simulink library "SUB_ECU_L4_MABX"  (R2018a)
settings: Solver=VariableStepAuto  StartTime=0.0  StopTime=10.0  RelTol=1e-3
libraries: EmE_MBD_Blockset x76, simulink x14, SUB_L4_Task_10000ms x1, SUB_L4_Task_1000ms x1, SUB_L4_Task_100ms x1, SUB_L4_Task_10ms_SUB_APTC x1, PTC_MBDS_LIB x1, SUB_L4_Task_10ms_SUB_BRKPEDARB x1, SUB_L4_Task_10ms_SUB_FAULT_MANAGER x1, SUB_L4_Task_10ms_SUB_STATE_CONTROL x1, SUB_L4_Task_10ms_SUB_STEERCTRL x1, simulink_need_slupdate x1
(part 1 of 2)
settings Model: Creator=Chris.Balton  LastModifiedBy=Gavin.Coelho

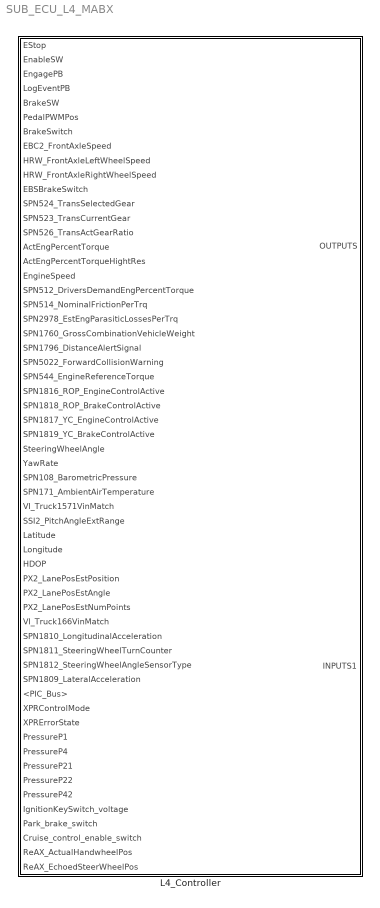
== system SUB_ECU_L4_MABX ==
  L4_Controller : Subsystem

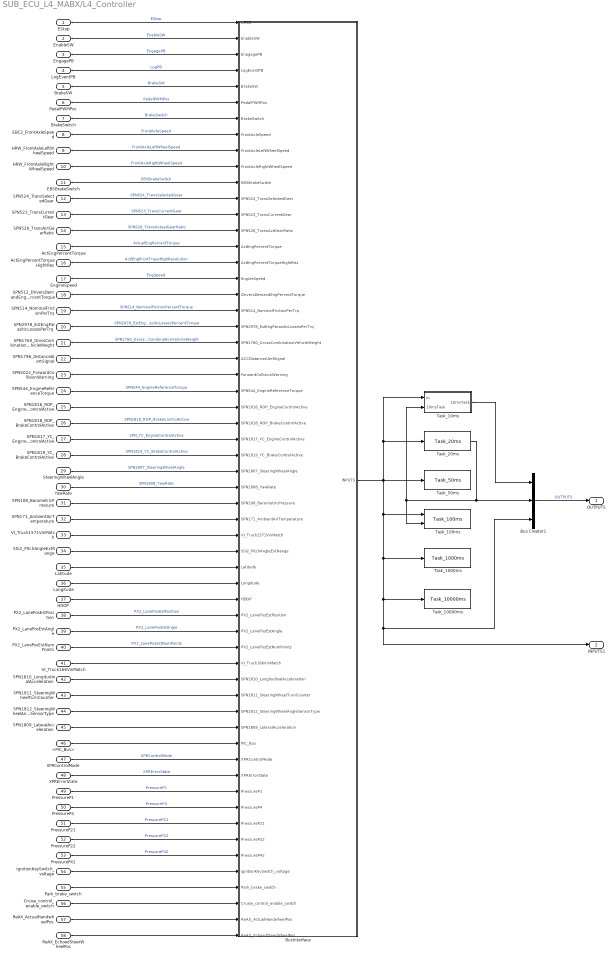
== system SUB_ECU_L4_MABX/L4_Controller ==
  EStop : Inport
  EnableSW : Inport  Port=2
  EngagePB : Inport  Port=3
  LogEventPB : Inport  Port=4
  BrakeSW : Inport  Port=5
  PedalPWMPos : Inport  Port=6
  BrakeSwitch : Inport  Port=7
  EBC2_FrontAxleSpeed : Inport  Port=8
  HRW_FrontAxleLeftWheelSpeed : Inport  Port=9
  HRW_FrontAxleRightWheelSpeed : Inport  Port=10
  EBSBrakeSwitch : Inport  Port=11
  SPN524_TransSelectedGear : Inport  Port=12
  SPN523_TransCurrentGear : Inport  Port=13
  SPN526_TransActGearRatio : Inport  Port=14
  ActEngPercentTorque : Inport  Port=15
  ActEngPercentTorqueHightRes : Inport  Port=16
  EngineSpeed : Inport  Port=17
  SPN512_DriversDemandEngPercentTorque : Inport  Port=18
  SPN514_NominalFrictionPerTrq : Inport  Port=19
  SPN2978_EstEngParasiticLossesPerTrq : Inport  Port=20
  SPN1760_GrossCombinationVehicleWeight : Inport  Port=21
  SPN1796_DistanceAlertSignal : Inport  Port=22
  SPN5022_ForwardCollisionWarning : Inport  Port=23
  SPN544_EngineReferenceTorque : Inport  Port=24
  SPN1816_ROP_EngineControlActive : Inport  Port=25
  SPN1818_ROP_BrakeControlActive : Inport  Port=26
  SPN1817_YC_EngineControlActive : Inport  Port=27
  SPN1819_YC_BrakeControlActive : Inport  Port=28
  SteeringWheelAngle : Inport  Port=29
  YawRate : Inport  Port=30
  SPN108_BarometricPressure : Inport  Port=31
  SPN171_AmbientAirTemperature : Inport  Port=32
  VI_Truck1571VinMatch : Inport  Port=33
  SSI2_PitchAngleExtRange : Inport  Port=34
  Latitude : Inport  Port=35
  Longitude : Inport  Port=36
  HDOP : Inport  Port=37
  PX2_LanePosEstPosition : Inport  Port=38
  PX2_LanePosEstAngle : Inport  Port=39
  PX2_LanePosEstNumPoints : Inport  Port=40
  VI_Truck166VinMatch : Inport  Port=41
  SPN1810_LongitudinalAcceleration : Inport  Port=42
  SPN1811_SteeringWheelTurnCounter : Inport  Port=43
  SPN1812_SteeringWheelAngleSensorType : Inport  Port=44
  SPN1809_LateralAcceleration : Inport  Port=45
  <PIC_Bus> : Inport  Port=46
  XPRControlMode : Inport  Port=47
  XPRErrorState : Inport  Port=48
  PressureP1 : Inport  Port=49
  PressureP4 : Inport  Port=50
  PressureP21 : Inport  Port=51
  PressureP22 : Inport  Port=52
  PressureP42 : Inport  Port=53
  IgnitionKeySwitch_voltage : Inport  Port=54
  Park_brake_switch : Inport  Port=55
  Cruise_control_enable_switch : Inport  Port=56
  ReAX_ActualHandwheelPos : Inport  Port=57
  ReAX_EchoedSteerWheelPos : Inport  Port=58
  Bus Creator1 : BusCreator  Inputs=3
  BusInterface : Subsystem
  Task_10000ms : SUB_L4_Task_10000ms/Task_10000ms
  Task_1000ms : SUB_L4_Task_1000ms/Task_1000ms
  Task_100ms : SUB_L4_Task_100ms/Task_100ms
  Task_10ms : Subsystem  TreatAsAtomicUnit=on  SystemSampleTime=0.01
  Task_20ms : SUB_L4_Task_20ms/Task_20ms
  Task_50ms : SUB_L4_Task_50ms/Task_50ms
  OUTPUTS : Outport
  INPUTS1 : Outport  Port=2
  wires:
  BrakeSW/1 -> BusInterface/5(BrakeSW)  "BrakeSW"
  ReAX_EchoedSteerWheelPos/1 -> BusInterface/58(ReAX_EchoedSteerWheelPos)
  ReAX_ActualHandwheelPos/1 -> BusInterface/57(ReAX_ActualHandwheelPos)
  EngagePB/1 -> BusInterface/3(EnagagePB)  "EngagePB"
  SPN1809_LateralAcceleration/1 -> BusInterface/45(SPN1809_LateralAcceleration)
  XPRErrorState/1 -> BusInterface/48(XPRErrorState)  "XPRErrorState"
  PressureP1/1 -> BusInterface/49(PressureP1)  "PressureP1"
  PressureP4/1 -> BusInterface/50(PressureP4)  "PressureP4"
  PressureP21/1 -> BusInterface/51(PressureP21)  "PressureP21"
  EBC2_FrontAxleSpeed/1 -> BusInterface/8(FrontAxleSpeed)  "FrontAxleSpeed"
  Task_10ms/1(10msTask) -> Bus Creator1/1
  EngineSpeed/1 -> BusInterface/17(EngineSpeed)  "EngSpeed"
  Cruise_control_enable_switch/1 -> BusInterface/56(Cruise_control_enable_switch)
  Longitude/1 -> BusInterface/36(Longitude)
  SPN5022_ForwardCollisionWarning/1 -> BusInterface/23(ForwardCollisionWarning)
  VI_Truck1571VinMatch/1 -> BusInterface/33(VI_Truck1571VinMatch)
  SPN512_DriversDemandEngPercentTorque/1 -> BusInterface/18(DriversDemandEngPercentTorque)
  Task_20ms/1 -> Bus Creator1/2, Task_100ms/2, Task_10ms/2(20msTask)
  SPN171_AmbientAirTemperature/1 -> BusInterface/32(SPN171_AmbientAirTemperature)
  SPN544_EngineReferenceTorque/1 -> BusInterface/24(SPN544_EngineReferenceTorque)  "SPN544_EngineReferenceTorque"
  HRW_FrontAxleRightWheelSpeed/1 -> BusInterface/10(FrontAxleRightWheelSpeed)  "FrontAxleRightWheelSpeed"
  SPN108_BarometricPressure/1 -> BusInterface/31(SPN108_BarometricPressure)
  PedalPWMPos/1 -> BusInterface/6(PedalPWMPos)  "PedalPWMPos"
  SPN524_TransSelectedGear/1 -> BusInterface/12(SPN524_TransSelectedGear)  "SPN524_TransSelectedGear"
  SPN1796_DistanceAlertSignal/1 -> BusInterface/22(ACCDistanceAlertSignal)
  Bus Creator1/1 -> OUTPUTS/1  "OUTPUTS"
  SPN1819_YC_BrakeControlActive/1 -> BusInterface/28(SPN1819_YC_BrakeControlActive)  "SPN1819_YC_BrakeControlActive"
  ActEngPercentTorque/1 -> BusInterface/15(ActEngPercentTorque)  "ActualEngPercentTorque"
  XPRControlMode/1 -> BusInterface/47(XPRControlMode)  "XPRControlMode"
  SSI2_PitchAngleExtRange/1 -> BusInterface/34(SSI2_PitchAngleExtRange)
  IgnitionKeySwitch_voltage/1 -> BusInterface/54(IgnitionKeySwitch_voltage)
  BrakeSwitch/1 -> BusInterface/7(BrakeSwitch)  "BrakeSwitch"
  HRW_FrontAxleLeftWheelSpeed/1 -> BusInterface/9(FrontAxleLeftWheelSpeed)  "FrontAxleLeftWheelSpeed"
  BusInterface/1(INPUTS) -> Task_50ms/1, Task_20ms/1, Task_10ms/1(In), Task_100ms/1, Task_1000ms/1, Task_10000ms/1, Bus Creator1/3, INPUTS1/1
  Park_brake_switch/1 -> BusInterface/55(Park_brake_switch)
  <PIC_Bus>/1 -> BusInterface/46(PIC_Bus)
  Latitude/1 -> BusInterface/35(Latitude)
  PressureP22/1 -> BusInterface/52(PressureP22)  "PressureP22"
  PressureP42/1 -> BusInterface/53(PressureP42)  "PressureP42"
  PX2_LanePosEstPosition/1 -> BusInterface/38(PX2_LanePosEstPosition)  "PX2_LanePosEstPosition"
  SPN514_NominalFrictionPerTrq/1 -> BusInterface/19(SPN514_NominalFrictionPerTrq)  "SPN514_NominalFrictionPercentTorque"
  SteeringWheelAngle/1 -> BusInterface/29(SPN1807_SteeringWheelAngle)  "SPN1807_SteeringWheelAngle"
  HDOP/1 -> BusInterface/37(HDOP)
  YawRate/1 -> BusInterface/30(SPN1808_YawRate)  "SPN1808_YawRate"
  EBSBrakeSwitch/1 -> BusInterface/11(EBSBrakeSwitch)  "EBSBrakeSwitch"
  SPN1811_SteeringWheelTurnCounter/1 -> BusInterface/43(SPN1811_SteeringWheelTurnCounter)
  SPN1760_GrossCombinationVehicleWeight/1 -> BusInterface/21(SPN1760_GrossCombinationVehicleWeight)  "SPN1760_GrossCombinationVehicleWeight"
  SPN2978_EstEngParasiticLossesPerTrq/1 -> BusInterface/20(SPN2978_EstEngParasiticLossesPerTrq)  "SPN2978_EstEngParasiticLossesPercentTorque"
  SPN1812_SteeringWheelAngleSensorType/1 -> BusInterface/44(SPN1812_SteeringWheelAngleSensorType)
  SPN526_TransActGearRatio/1 -> BusInterface/14(SPN526_TransActGearRatio)  "SPN526_TransActualGearRatio"
  SPN1818_ROP_BrakeControlActive/1 -> BusInterface/26(SPN1818_ROP_BrakeControlActive)  "SPN1818_ROP_BrakeControlActive"
  PX2_LanePosEstAngle/1 -> BusInterface/39(PX2_LanePosEstAngle)  "PX2_LanePosEstAngle"
  ActEngPercentTorqueHightRes/1 -> BusInterface/16(ActEngPercentTorqueHightRes)  "ActlEngPrcntTrqueHighResolution"
  SPN1810_LongitudinalAcceleration/1 -> BusInterface/42(SPN1810_LongitudinalAcceleration)
  PX2_LanePosEstNumPoints/1 -> BusInterface/40(PX2_LanePosEstNumPoints)  "PX2_LanePosEstNumPoints"
  EStop/1 -> BusInterface/1(Estop)  "EStop"
  VI_Truck166VinMatch/1 -> BusInterface/41(VI_Truck166VinMatch)
  SPN523_TransCurrentGear/1 -> BusInterface/13(SPN523_TransCurrentGear)  "SPN523_TransCurrentGear"
  SPN1817_YC_EngineControlActive/1 -> BusInterface/27(SPN1817_YC_EngineControlActive)  "SPN_YC_EngineControlActive"
  EnableSW/1 -> BusInterface/2(EnableSW)  "EnableSW"
  SPN1816_ROP_EngineControlActive/1 -> BusInterface/25(SPN1816_ROP_EngineControlActive)
  LogEventPB/1 -> BusInterface/4(LogEventPB)  "LogPB"

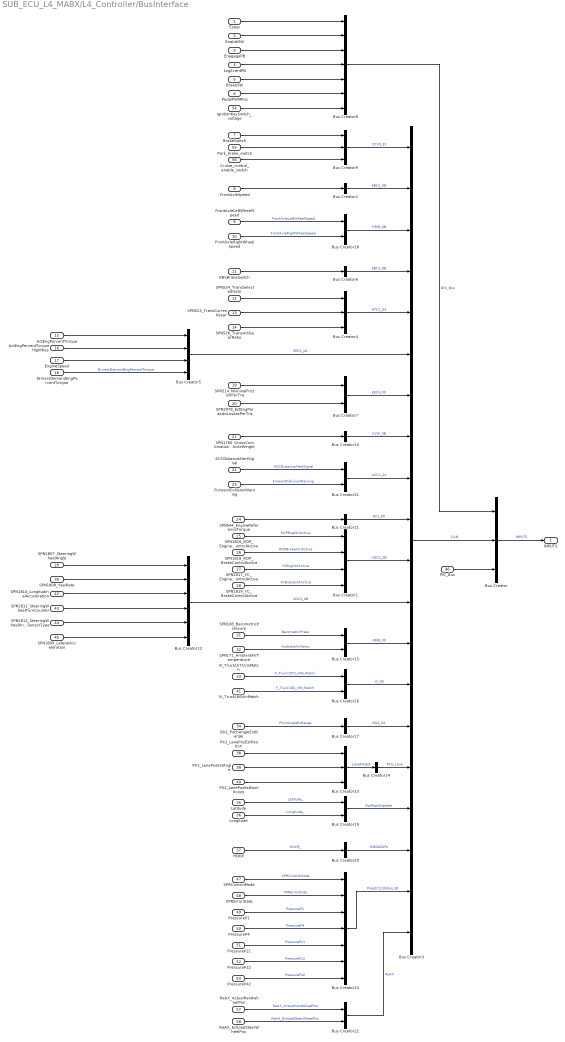
== system SUB_ECU_L4_MABX/L4_Controller/BusInterface ==
  Estop : Inport
  EnableSW : Inport  Port=2
  EnagagePB : Inport  Port=3
  LogEventPB : Inport  Port=4
  BrakeSW : Inport  Port=5
  PedalPWMPos : Inport  Port=6
  BrakeSwitch : Inport  Port=7
  FrontAxleSpeed : Inport  Port=8
  FrontAxleLeftWheelSpeed : Inport  Port=9
  FrontAxleRightWheelSpeed : Inport  Port=10
  EBSBrakeSwitch : Inport  Port=11
  SPN524_TransSelectedGear : Inport  Port=12
  SPN523_TransCurrentGear : Inport  Port=13
  SPN526_TransActGearRatio : Inport  Port=14
  ActEngPercentTorque : Inport  Port=15
  ActEngPercentTorqueHightRes : Inport  Port=16
  EngineSpeed : Inport  Port=17
  DriversDemandEngPercentTorque : Inport  Port=18
  SPN514_NominalFrictionPerTrq : Inport  Port=19
  SPN2978_EstEngParasiticLossesPerTrq : Inport  Port=20
  SPN1760_GrossCombinationVehicleWeight : Inport  Port=21
  ACCDistanceAlertSignal : Inport  Port=22
  ForwardCollisionWarning : Inport  Port=23
  SPN544_EngineReferenceTorque : Inport  Port=24
  SPN1816_ROP_EngineControlActive : Inport  Port=25
  SPN1818_ROP_BrakeControlActive : Inport  Port=26
  SPN1817_YC_EngineControlActive : Inport  Port=27
  SPN1819_YC_BrakeControlActive : Inport  Port=28
  SPN1807_SteeringWheelAngle : Inport  Port=29
  SPN1808_YawRate : Inport  Port=30
  SPN108_BarometricPressure : Inport  Port=31
  SPN171_AmbientAirTemperature : Inport  Port=32
  VI_Truck1571VinMatch : Inport  Port=33
  SSI2_PitchAngleExtRange : Inport  Port=34
  Latitude : Inport  Port=35
  Longitude : Inport  Port=36
  HDOP : Inport  Port=37
  PX2_LanePosEstPosition : Inport  Port=38
  PX2_LanePosEstAngle : Inport  Port=39
  PX2_LanePosEstNumPoints : Inport  Port=40
  VI_Truck166VinMatch : Inport  Port=41
  SPN1810_LongitudinalAcceleration : Inport  Port=42
  SPN1811_SteeringWheelTurnCounter : Inport  Port=43
  SPN1812_SteeringWheelAngleSensorType : Inport  Port=44
  SPN1809_LateralAcceleration : Inport  Port=45
  PIC_Bus : Inport  Port=46
  XPRControlMode : Inport  Port=47
  XPRErrorState : Inport  Port=48
  PressureP1 : Inport  Port=49
  PressureP4 : Inport  Port=50
  PressureP21 : Inport  Port=51
  PressureP22 : Inport  Port=52
  PressureP42 : Inport  Port=53
  IgnitionKeySwitch_voltage : Inport  Port=54
  Park_brake_switch : Inport  Port=55
  Cruise_control_enable_switch : Inport  Port=56
  ReAX_ActualHandwheelPos : Inport  Port=57
  ReAX_EchoedSteerWheelPos : Inport  Port=58
  Bus Creator{,4,9,13} (4 alike) : BusCreator  Inputs=3
  Bus Creator1 : BusCreator  Inputs=4
  Bus Creator{2,6,10..11,14,17,20} (7 alike) : BusCreator  Inputs=1
  Bus Creator12 : BusCreator  Inputs=6
  Bus Creator{7,15..16,18..19,21..22} (7 alike) : BusCreator  Inputs=2
  Bus Creator23 : BusCreator  Inputs=7
  Bus Creator3 : BusCreator  Inputs=20
  Bus Creator5 : BusCreator  Inputs=4
  Bus Creator8 : BusCreator  Inputs=7
  INPUTS : Outport
  wires:
  BrakeSW/1 -> Bus Creator8/5
  Bus Creator22/1 -> Bus Creator3/20  "ReAX"
  ReAX_ActualHandwheelPos/1 -> Bus Creator22/1  "ReAX_ActualHandwheelPos"
  ReAX_EchoedSteerWheelPos/1 -> Bus Creator22/2  "ReAX_EchoedSteerWheelPos"
  Bus Creator23/1 -> Bus Creator3/19  "Prop2C2_Status_30"
  XPRControlMode/1 -> Bus Creator23/1  "XPRControlMode"
  PressureP21/1 -> Bus Creator23/5  "PressureP21"
  XPRErrorState/1 -> Bus Creator23/2  "XPRErrorState"
  PressureP42/1 -> Bus Creator23/7  "PressureP42"
  PressureP1/1 -> Bus Creator23/3  "PressureP1"
  PressureP22/1 -> Bus Creator23/6  "PressureP22"
  PressureP4/1 -> Bus Creator23/4  "PressureP4"
  SPN1809_LateralAcceleration/1 -> Bus Creator12/6
  SPN1812_SteeringWheelAngleSensorType/1 -> Bus Creator12/5
  SPN1811_SteeringWheelTurnCounter/1 -> Bus Creator12/4
  SPN1810_LongitudinalAcceleration/1 -> Bus Creator12/3
  VI_Truck166VinMatch/1 -> Bus Creator16/2  "F_Truck166_VIN_Match"
  Bus Creator1/1 -> Bus Creator3/11  "VDC1_0B"
  SPN1819_YC_BrakeControlActive/1 -> Bus Creator1/4  "YCBrakeCtrlActive"
  SPN1817_YC_EngineControlActive/1 -> Bus Creator1/3  "YCEngCtrlActive"
  SPN1818_ROP_BrakeControlActive/1 -> Bus Creator1/2  "ROPBrakeCtrlActive"
  SPN1816_ROP_EngineControlActive/1 -> Bus Creator1/1  "ROPEngCtrlActive"
  SPN1808_YawRate/1 -> Bus Creator12/2
  Bus Creator/1 -> INPUTS/1  "INPUTS"
  EngineSpeed/1 -> Bus Creator5/3
  PX2_LanePosEstPosition/1 -> Bus Creator13/1
  FrontAxleSpeed/1 -> Bus Creator2/1
  SPN1807_SteeringWheelAngle/1 -> Bus Creator12/1
  Bus Creator14/1 -> Bus Creator3/16  "PX2_Lane"
  SPN526_TransActGearRatio/1 -> Bus Creator4/3
  SPN544_EngineReferenceTorque/1 -> Bus Creator11/1
  Bus Creator12/1 -> Bus Creator3/12  "VDC2_0B"
  Bus Creator6/1 -> Bus Creator3/4  "EBC1_0B"
  Bus Creator4/1 -> Bus Creator3/5  "ETC2_03"
  SPN2978_EstEngParasiticLossesPerTrq/1 -> Bus Creator7/2
  SPN514_NominalFrictionPerTrq/1 -> Bus Creator7/1
  SPN524_TransSelectedGear/1 -> Bus Creator4/1
  Bus Creator2/1 -> Bus Creator3/2  "EBC2_0B"
  SPN523_TransCurrentGear/1 -> Bus Creator4/2
  Bus Creator9/1 -> Bus Creator3/1  "CCVS_31"
  Bus Creator10/1 -> Bus Creator3/8  "CVW_0B"
  PX2_LanePosEstAngle/1 -> Bus Creator13/2
  SPN1760_GrossCombinationVehicleWeight/1 -> Bus Creator10/1
  Bus Creator7/1 -> Bus Creator3/7  "EEC3_00"
  ActEngPercentTorqueHightRes/1 -> Bus Creator5/2
  Bus Creator11/1 -> Bus Creator3/10  "EC1_00"
  EBSBrakeSwitch/1 -> Bus Creator6/1
  BrakeSwitch/1 -> Bus Creator9/1
  Bus Creator3/1 -> Bus Creator/2  "CAN"
  ActEngPercentTorque/1 -> Bus Creator5/1
  EnagagePB/1 -> Bus Creator8/3
  Bus Creator5/1 -> Bus Creator3/6  "EEC1_00"
  PX2_LanePosEstNumPoints/1 -> Bus Creator13/3
  Bus Creator8/1 -> Bus Creator/1  "DIO_Bus"
  Bus Creator13/1 -> Bus Creator14/1  "LanePosEst"
  SPN108_BarometricPressure/1 -> Bus Creator15/1  "BarometricPress"
  SPN171_AmbientAirTemperature/1 -> Bus Creator15/2  "AmbientAirTemp"
  VI_Truck1571VinMatch/1 -> Bus Creator16/1  "F_Truck1571_VIN_Match"
  SSI2_PitchAngleExtRange/1 -> Bus Creator17/1  "PitchAngleExRange"
  Bus Creator15/1 -> Bus Creator3/13  "AMB_00"
  Bus Creator16/1 -> Bus Creator3/14  "VI_00"
  Bus Creator17/1 -> Bus Creator3/15  "SSI2_03"
  PedalPWMPos/1 -> Bus Creator8/6
  FrontAxleLeftWheelSpeed/1 -> Bus Creator18/1  "FrontAxleLeftWheelSpeed"
  FrontAxleRightWheelSpeed/1 -> Bus Creator18/2  "FrontAxleRightWheelSpeed"
  Bus Creator18/1 -> Bus Creator3/3  "HRW_0B"
  Latitude/1 -> Bus Creator19/1  "Latitude_"
  Longitude/1 -> Bus Creator19/2  "Longitude_"
  Bus Creator19/1 -> Bus Creator3/17  "PosRapidUpdate"
  HDOP/1 -> Bus Creator20/1  "HDOP_"
  Bus Creator20/1 -> Bus Creator3/18  "GNSSDOPs"
  ACCDistanceAlertSignal/1 -> Bus Creator21/1  "ACCDistanceAlertSignal"
  ForwardCollisionWarning/1 -> Bus Creator21/2  "ForwardCollisionWarning"
  Bus Creator21/1 -> Bus Creator3/9  "ACC1_2A"
  DriversDemandEngPercentTorque/1 -> Bus Creator5/4  "DriversDemandEngPercentTorque"
  PIC_Bus/1 -> Bus Creator/3
  IgnitionKeySwitch_voltage/1 -> Bus Creator8/7
  Park_brake_switch/1 -> Bus Creator9/2
  Cruise_control_enable_switch/1 -> Bus Creator9/3
  EnableSW/1 -> Bus Creator8/2
  Estop/1 -> Bus Creator8/1
  LogEventPB/1 -> Bus Creator8/4

== system SUB_ECU_L4_MABX/L4_Controller/Task_10ms ==
  In : Inport
  20msTask : Inport  Port=2
  APTC_10ms : SUB_L4_Task_10ms_SUB_APTC/APTC_10ms
  AutonomousEnable : Subsystem
  BRKPEDARB_10ms : SUB_L4_Task_10ms_SUB_BRKPEDARB/BRKPEDARB_10ms
  Bus Creator : BusCreator  Inputs=6
  FAULT_MANAGER_10ms : SUB_L4_Task_10ms_SUB_FAULT_MANAGER/FAULT_MANAGER_10ms
  STATE_CONTROL_10ms : SUB_L4_Task_10ms_SUB_STATE_CONTROL/STATE_CONTROL_10ms
  STEERCTRL_10ms : SUB_L4_Task_10ms_SUB_STEERCTRL/STEERCTRL_10ms
  Vehicle_speed_target : Subsystem
  10msTask : Outport
  wires:
  In/1 -> AutonomousEnable/1(In)
  APTC_10ms/1 -> Bus Creator/2  "APTC"
  Bus Creator/1 -> 10msTask/1  "10msTask"
  STEERCTRL_10ms/1 -> STATE_CONTROL_10ms/3, BRKPEDARB_10ms/2, Bus Creator/1  "SteeringControl"
  STATE_CONTROL_10ms/1 -> Bus Creator/3, APTC_10ms/2  "StateControl"
  BRKPEDARB_10ms/1 -> STATE_CONTROL_10ms/2, Bus Creator/4  "BrakeCtrl"
  20msTask/1 -> Vehicle_speed_target/2(20msTask), STEERCTRL_10ms/1
  Vehicle_speed_target/1(SpeedTarget) -> BRKPEDARB_10ms/3, Bus Creator/5, STATE_CONTROL_10ms/4
  AutonomousEnable/1(Out) -> Vehicle_speed_target/1(In), FAULT_MANAGER_10ms/1, APTC_10ms/1, BRKPEDARB_10ms/1, STEERCTRL_10ms/2, STATE_CONTROL_10ms/1
  AutonomousEnable/2(AutonomousState) -> Bus Creator/6

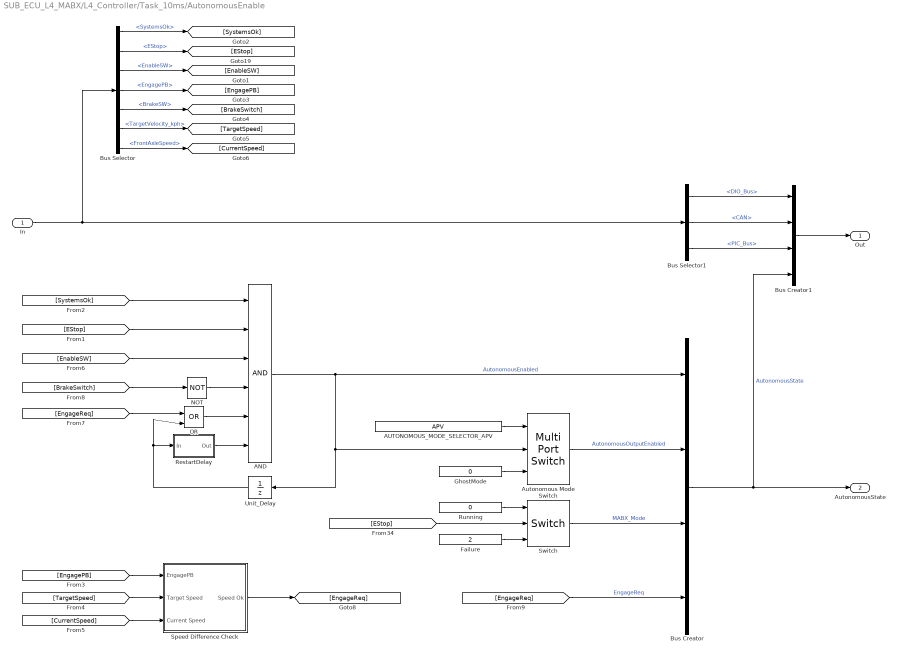
== system SUB_ECU_L4_MABX/L4_Controller/Task_10ms/AutonomousEnable ==
  In : Inport
  AND : Logic  Inputs=6  AllPortsSameDT=off  OutDataTypeStr=boolean
  AUTONOMOUS_MODE_SELECTOR_APV : EmE_MBD_Blockset/Sources/APV  conval=AUTONOMOUS_MODE_SELECTOR_APV
      settings: SourceProductName=PACCAR EmE MBD Blockset
  Autonomous Mode Switch : MultiPortSwitch  DataPortOrder=Specify indices  DataPortIndices={ENUM_AUTONOMOUS_MODE_T.AUTO,ENUM_AUTONOMOUS_MODE_T.GHOST}  DiagnosticForDefault=None
  Bus Creator : BusCreator  Inputs=4
  Bus Creator1 : BusCreator  Inputs=4
  Bus Selector : BusSelector  OutputSignals=PIC_Bus.SystemsOk,DIO_Bus.EStop,DIO_Bus.EnableSW,DIO_Bus.EngagePB,DIO_Bus.BrakeSW,PIC_Bus.TargetVelocity_kph,CAN.EBC2_0B.FrontAxleSpeed
  Bus Selector1 : BusSelector  OutputSignals=DIO_Bus,CAN,PIC_Bus
  Failure : Constant  Value=2  OutDataTypeStr=int8
  GhostMode : Constant  Value=0  OutDataTypeStr=int8
  NOT : Logic  Operator=NOT  IconShape=distinctive  AllPortsSameDT=off  OutDataTypeStr=boolean
  OR : Logic  Operator=OR  IconShape=distinctive  AllPortsSameDT=off  OutDataTypeStr=boolean
  RestartDelay : Subsystem
  Running : Constant  Value=0  OutDataTypeStr=int8
  Speed Difference Check : Subsystem
  Switch : PTC_MBDS_LIB/MBDS Standard Library/Signals & Systems/Signal Routing/Switch  OutDataTypeStr_=Inherit: Inherit via back propagation  SaturateOnIntegerOverflow_=on  InputSameDT_=on  PTC_MBDS_BlockVersion=5.41  PTC_BlockType=PTC_MBDS_Switch
      settings: SourceProductName=PACCAR Technical Center MBDS Library
  Unit_Delay : UnitDelay  SampleTime=-1
      settings: AttributesFormatString=IC: %<vinit>
  Out : Outport
  AutonomousState : Outport  Port=2
  wires:
  AND/1 -> Unit_Delay/1, Autonomous Mode Switch/2, Bus Creator/1  "AutonomousEnabled"
  In/1 -> Bus Selector/1, Bus Selector1/1
  Failure/1 -> Switch/3
  Running/1 -> Switch/1
  Switch/1 -> Bus Creator/3  "MABX_Mode"
  Bus Creator/1 -> Bus Creator1/4, AutonomousState/1  "AutonomousState"
  Bus Creator1/1 -> Out/1
  Bus Selector1/1 -> Bus Creator1/1  "<DIO_Bus>"
  Bus Selector1/2 -> Bus Creator1/2  "<CAN>"
  Bus Selector1/3 -> Bus Creator1/3  "<PIC_Bus>"
  Autonomous Mode Switch/1 -> Bus Creator/2  "AutonomousOutputEnabled"
  AUTONOMOUS_MODE_SELECTOR_APV/1 -> Autonomous Mode Switch/1
  GhostMode/1 -> Autonomous Mode Switch/3
  [EStop] -> Switch/2
  [EStop] -> AND/2
  Bus Selector/2 -> [EStop]  "<EStop>"
  Bus Selector/3 -> [EnableSW]  "<EnableSW>"
  [SystemsOk] -> AND/1
  [EngagePB] -> Speed Difference Check/1(EngagePB)
  Bus Selector/1 -> [SystemsOk]  "<SystemsOk>"
  Bus Selector/4 -> [EngagePB]  "<EngagePB>"
  Bus Selector/5 -> [BrakeSwitch]  "<BrakeSW>"
  Bus Selector/6 -> [TargetSpeed]  "<TargetVelocity_kph>"
  Bus Selector/7 -> [CurrentSpeed]  "<FrontAxleSpeed>"
  [TargetSpeed] -> Speed Difference Check/2(Target Speed)
  [CurrentSpeed] -> Speed Difference Check/3(Current Speed)
  [EnableSW] -> AND/3
  [EngageReq] -> OR/1
  Speed Difference Check/1(Speed Ok) -> [EngageReq]
  [BrakeSwitch] -> NOT/1
  NOT/1 -> AND/4
  OR/1 -> AND/5
  [EngageReq] -> Bus Creator/4  "EngageReq"
  Unit_Delay/1 -> OR/2, RestartDelay/1(In)
  RestartDelay/1(Out) -> AND/6

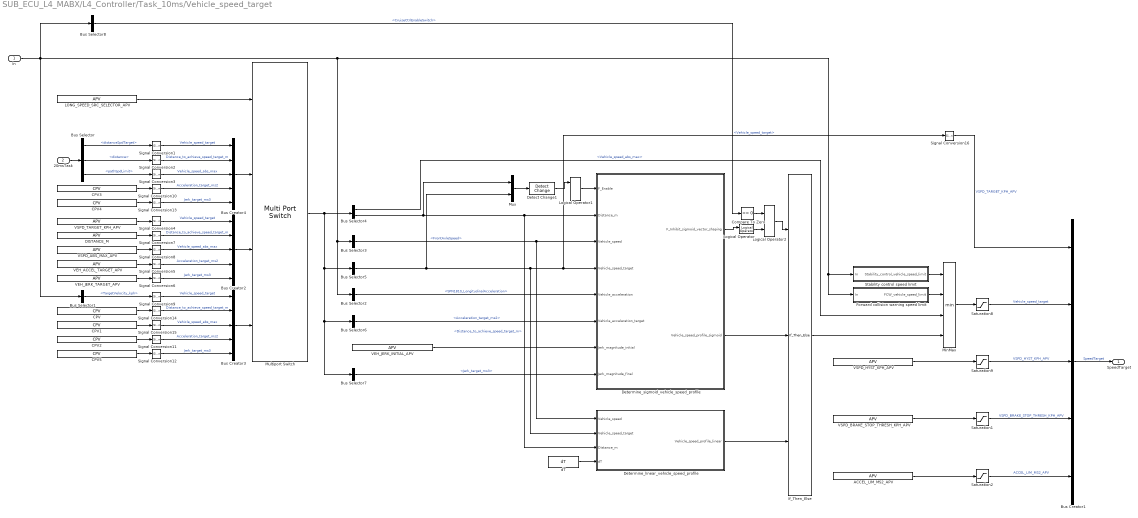
== system SUB_ECU_L4_MABX/L4_Controller/Task_10ms/Vehicle_speed_target ==
  In : Inport
  20msTask : Inport  Port=2
  ACCEL_LIM_MS2_APV : EmE_MBD_Blockset/Sources/APV  conval=-5
      settings: SourceProductName=PACCAR EmE MBD Blockset
  Bus Creator{1..4} (4 alike) : BusCreator  Inputs=5
  Bus Selector : BusSelector  OutputSignals=mapping.distanceSpdTarget,mapping.distance,mapping.pathSpdLimit
  Bus Selector1 : BusSelector  OutputSignals=PIC_Bus.TargetVelocity_kph
  Bus Selector2 : BusSelector  OutputSignals=CAN.VDC2_0B.SPN1810_LongitudinalAcceleration
  Bus Selector3 : BusSelector  OutputSignals=CAN.EBC2_0B.FrontAxleSpeed
  Bus Selector4 : BusSelector  OutputSignals=Vehicle_speed_abs_max,Distance_to_achieve_speed_target_m
  Bus Selector5 : BusSelector  OutputSignals=Vehicle_speed_target
  Bus Selector6 : BusSelector  OutputSignals=Acceleration_target_ms2
  Bus Selector7 : BusSelector  OutputSignals=Jerk_target_ms3
  Bus Selector8 : BusSelector  OutputSignals=CAN.CCVS_31.CruiseCtrlEnableSwitch
  CPV{,2..4} (4 alike) : EmE_MBD_Blockset/Sources/CPV  conval=0
      settings: SourceProductName=PACCAR EmE MBD Blockset
  CPV1 : EmE_MBD_Blockset/Sources/CPV  conval=255
      settings: SourceProductName=PACCAR EmE MBD Blockset
  CPV5 : EmE_MBD_Blockset/Sources/CPV  conval=0.5
      settings: SourceProductName=PACCAR EmE MBD Blockset
  Compare To Zero : simulink/Logic and Bit Operations/Compare To Zero  relop===  OutDataTypeStr=boolean
  DISTANCE_M : EmE_MBD_Blockset/Sources/APV  conval=DISTANCE_M
      settings: SourceProductName=PACCAR EmE MBD Blockset
  Detect Change1 : simulink/Logic and Bit Operations/Detect Change  vinit=0  InputProcessing=Inherited  OutDataTypeStr=boolean
      settings: AttributesFormatString=IC: %<vinit>
  Determine_linear_vehicle_speed_profile : Subsystem
  Determine_sigmoid_vehicle_speed_profile : Subsystem
  Forward collision warning speed limit : Subsystem
  If_Then_Else : EmE_MBD_Blockset/Signal Routing/If_Then_Else
      settings: SourceProductName=PACCAR EmE MBD Blockset
  LONG_SPEED_SRC_SELECTOR_APV : EmE_MBD_Blockset/Sources/APV  conval=LONG_SPEED_SRC_SELECTOR_APV
      settings: SourceProductName=PACCAR EmE MBD Blockset
  Logical Operator : EmE_MBD_Blockset/Logic and Bit Operations/Logical Operator  Operator=NOT  Inputs=2
      settings: SourceProductName=PACCAR EmE MBD Blockset
  Logical Operator1 : EmE_MBD_Blockset/Logic and Bit Operations/Logical Operator  Operator=OR  Inputs=1
      settings: SourceProductName=PACCAR EmE MBD Blockset
  Logical Operator2 : EmE_MBD_Blockset/Logic and Bit Operations/Logical Operator  Operator=AND  Inputs=2
      settings: SourceProductName=PACCAR EmE MBD Blockset
  MinMax : MinMax  Inputs=4  InputSameDT=on
  Multiport Switch : MultiPortSwitch  DataPortOrder=Specify indices  DataPortIndices={ENUM_LONG_SPEED_DEMAND_SOURCE_T.GPS_PATH,ENUM_LONG_SPEED_DEMAND_SOURCE_T.OVERRIDE,ENUM_LONG_SPEED_DEMAND_SOURCE_T.WAYPOINTS}  DiagnosticForDefault=None
  Mux : Mux  Inputs=2
  Saturation1 : Saturate  UpperLimit=5  LowerLimit=0
      settings: AttributesFormatString=|
      | Min: %<LowerLimit>
      | Max: %<UpperLimit>
  Saturation2 : Saturate  UpperLimit=15.562  LowerLimit=-15.562
      settings: AttributesFormatString=|
      | Min: %<LowerLimit>
      | Max: %<UpperLimit>
  Saturation8 : Saturate  UpperLimit=100  LowerLimit=0
      settings: AttributesFormatString=|
      | Min: %<LowerLimit>
      | Max: %<UpperLimit>
  Saturation9 : Saturate  UpperLimit=5  LowerLimit=0
      settings: AttributesFormatString=|
      | Min: %<LowerLimit>
      | Max: %<UpperLimit>
  Signal Conversion{1..16} (16 alike) : SignalConversion  OverrideOpt=off
  Stability control speed limit : Subsystem
  VEH_ACCEL_TARGET_APV : EmE_MBD_Blockset/Sources/APV  conval=-0.5
      settings: SourceProductName=PACCAR EmE MBD Blockset
  VEH_JERK_INITIAL_APV : EmE_MBD_Blockset/Sources/APV  conval=0.4
      settings: SourceProductName=PACCAR EmE MBD Blockset
  VEH_JERK_TARGET_APV : EmE_MBD_Blockset/Sources/APV  conval=0.2
      settings: SourceProductName=PACCAR EmE MBD Blockset
  VSPD_ABS_MAX_APV : EmE_MBD_Blockset/Sources/APV  conval=255
      settings: SourceProductName=PACCAR EmE MBD Blockset
  VSPD_BRAKE_STOP_THRESH_KPH_APV : EmE_MBD_Blockset/Sources/APV  conval=2
      settings: SourceProductName=PACCAR EmE MBD Blockset
  VSPD_HYST_KPH_APV : EmE_MBD_Blockset/Sources/APV  conval=1
      settings: SourceProductName=PACCAR EmE MBD Blockset
  VSPD_TARGET_KPH_APV : EmE_MBD_Blockset/Sources/APV  conval=VSPD_TARGET_KPH_APV
      settings: SourceProductName=PACCAR EmE MBD Blockset
  dT : EmE_MBD_Blockset/Sources/dT
      settings: SourceProductName=PACCAR EmE MBD Blockset
  SpeedTarget : Outport
  wires:
  In/1 -> Bus Selector1/1, Bus Selector2/1, Bus Selector3/1, Stability control speed limit/1(In), Forward collision warning speed limit/1(In), Bus Selector8/1
  VSPD_HYST_KPH_APV/1 -> Saturation9/1
  Saturation8/1 -> Bus Creator1/2  "Vehicle_speed_target"
  Stability control speed limit/1(Stability_control_vehicle_speed_limit) -> MinMax/1
  LONG_SPEED_SRC_SELECTOR_APV/1 -> Multiport Switch/1
  Saturation1/1 -> Bus Creator1/4  "VSPD_BRAKE_STOP_THRESH_KPH_APV"
  MinMax/1 -> Saturation8/1
  VSPD_BRAKE_STOP_THRESH_KPH_APV/1 -> Saturation1/1
  ACCEL_LIM_MS2_APV/1 -> Saturation2/1
  Bus Selector1/1 -> Signal Conversion9/1  "<TargetVelocity_kph>"
  Saturation2/1 -> Bus Creator1/5  "ACCEL_LIM_MS2_APV"
  Saturation9/1 -> Bus Creator1/3  "VSPD_HYST_KPH_APV"
  Bus Creator1/1 -> SpeedTarget/1  "SpeedTarget"
  Determine_linear_vehicle_speed_profile/1(Vehicle_speed_profile_linear) -> If_Then_Else/3
  Determine_sigmoid_vehicle_speed_profile/1(F_Inhibit_sigmoid_vector_shaping) -> Logical Operator/1
  Bus Selector2/1 -> Determine_sigmoid_vehicle_speed_profile/5(Vehicle_acceleration)  "<SPN1810_LongitudinalAcceleration>"
  dT/1 -> Determine_linear_vehicle_speed_profile/4(dT)
  Logical Operator1/1 -> Determine_sigmoid_vehicle_speed_profile/1(F_Enable)
  Bus Selector3/1 -> Determine_sigmoid_vehicle_speed_profile/3(Vehicle_speed), Determine_linear_vehicle_speed_profile/1(Vehicle_speed)  "<FrontAxleSpeed>"
  Bus Selector4/2 -> Determine_sigmoid_vehicle_speed_profile/2(Distance_m), Determine_linear_vehicle_speed_profile/3(Distance_m), Mux/1  "<Distance_to_achieve_speed_target_m>"
  Logical Operator/1 -> Logical Operator2/2
  Bus Selector6/1 -> Determine_sigmoid_vehicle_speed_profile/6(Vehicle_acceleration_target)  "<Acceleration_target_ms2>"
  Bus Selector/2 -> Signal Conversion2/1  "<distance>"
  20msTask/1 -> Bus Selector/1
  If_Then_Else/1 -> MinMax/4
  Bus Creator4/1 -> Multiport Switch/2
  VSPD_TARGET_KPH_APV/1 -> Signal Conversion4/1
  DISTANCE_M/1 -> Signal Conversion7/1
  Bus Selector/1 -> Signal Conversion1/1  "<distanceSpdTarget>"
  Bus Selector/3 -> Signal Conversion3/1  "<pathSpdLimit>"
  VSPD_ABS_MAX_APV/1 -> Signal Conversion8/1
  CPV/1 -> Signal Conversion14/1
  CPV1/1 -> Signal Conversion15/1
  Multiport Switch/1 -> Bus Selector7/1, Bus Selector6/1, Bus Selector5/1, Bus Selector4/1
  Signal Conversion3/1 -> Bus Creator4/3  "Vehicle_speed_abs_max"
  Signal Conversion2/1 -> Bus Creator4/2  "Distance_to_achieve_speed_target_m"
  Signal Conversion1/1 -> Bus Creator4/1  "Vehicle_speed_target"
  Signal Conversion10/1 -> Bus Creator4/4  "Acceleration_target_ms2"
  CPV2/1 -> Signal Conversion11/1
  CPV3/1 -> Signal Conversion10/1
  Bus Selector4/1 -> MinMax/3  "<Vehicle_speed_abs_max>"
  Forward collision warning speed limit/1(FCW_vehicle_speed_limit) -> MinMax/2
  Detect Change1/1 -> Logical Operator1/1
  Mux/1 -> Detect Change1/1
  Bus Selector5/1 -> Determine_linear_vehicle_speed_profile/2(Vehicle_speed_target), Signal Conversion16/1, Determine_sigmoid_vehicle_speed_profile/4(Vehicle_speed_target), Mux/2  "<Vehicle_speed_target>"
  Determine_sigmoid_vehicle_speed_profile/2(Vehicle_speed_profile_sigmoid) -> If_Then_Else/2
  CPV4/1 -> Signal Conversion13/1
  Signal Conversion13/1 -> Bus Creator4/5  "Jerk_target_ms3"
  Signal Conversion6/1 -> Bus Creator2/5  "Jerk_target_ms3"
  Signal Conversion5/1 -> Bus Creator2/4  "Acceleration_target_ms2"
  Signal Conversion4/1 -> Bus Creator2/1  "Vehicle_speed_target"
  Signal Conversion7/1 -> Bus Creator2/2  "Distance_to_achieve_speed_target_m"
  Signal Conversion8/1 -> Bus Creator2/3  "Vehicle_speed_abs_max"
  Bus Creator2/1 -> Multiport Switch/3
  VEH_ACCEL_TARGET_APV/1 -> Signal Conversion5/1
  VEH_JERK_TARGET_APV/1 -> Signal Conversion6/1
  Bus Creator3/1 -> Multiport Switch/4
  Signal Conversion15/1 -> Bus Creator3/3  "Vehicle_speed_abs_max"
  Signal Conversion14/1 -> Bus Creator3/2  "Distance_to_achieve_speed_target_m"
  Signal Conversion9/1 -> Bus Creator3/1  "Vehicle_speed_target"
  Signal Conversion11/1 -> Bus Creator3/4  "Acceleration_target_ms2"
  Signal Conversion12/1 -> Bus Creator3/5  "Jerk_target_ms3"
  CPV5/1 -> Signal Conversion12/1
  Bus Selector7/1 -> Determine_sigmoid_vehicle_speed_profile/8(Jerk_magnitude_final)  "<Jerk_target_ms3>"
  VEH_JERK_INITIAL_APV/1 -> Determine_sigmoid_vehicle_speed_profile/7(Jerk_magnitude_initial)
  Logical Operator2/1 -> If_Then_Else/1
  Bus Selector8/1 -> Compare To Zero/1  "<CruiseCtrlEnableSwitch>"
  Compare To Zero/1 -> Logical Operator2/1
  Signal Conversion16/1 -> Bus Creator1/1  "VSPD_TARGET_KPH_APV"

== system SUB_ECU_L4_MABX/L4_Controller/Task_10ms/AutonomousEnable/RestartDelay ==
  In : Inport
  2000ms Delay : Constant  Value=2000  OutDataTypeStr=uint16
  Delay : Subsystem
  Detect Fall Nonpositive : simulink/Logic and Bit Operations/Detect Fall Nonpositive  vinit=0  OutDataTypeStr=boolean
      settings: SourceProductName=Simulink  SourceProductBaseCode=SL
  NOT1 : Logic  Operator=NOT  IconShape=distinctive  AllPortsSameDT=off  OutDataTypeStr=boolean
  Out : Outport
  wires:
  Detect Fall Nonpositive/1 -> Delay/1(In)
  In/1 -> Detect Fall Nonpositive/1
  Delay/1(out) -> NOT1/1
  2000ms Delay/1 -> Delay/2(time_ms)
  NOT1/1 -> Out/1

== system SUB_ECU_L4_MABX/L4_Controller/Task_10ms/AutonomousEnable/Speed Difference Check ==
  EngagePB : Inport
  Target Speed : Inport  Port=2
  Current Speed : Inport  Port=3
  AND : Logic  IconShape=distinctive  AllPortsSameDT=off  OutDataTypeStr=boolean
  Compare To Constant : simulink/Logic and Bit Operations/Compare To Constant  relop=>=  const=-5  OutDataTypeStr=boolean
  Subtract : Sum  Inputs=+-  InputSameDT=on
  Speed Ok : Outport
  wires:
  Current Speed/1 -> Subtract/2
  Subtract/1 -> Compare To Constant/1
  AND/1 -> Speed Ok/1
  Compare To Constant/1 -> AND/2
  Target Speed/1 -> Subtract/1
  EngagePB/1 -> AND/1

== system SUB_ECU_L4_MABX/L4_Controller/Task_10ms/Vehicle_speed_target/Determine_linear_vehicle_speed_profile ==
  Vehicle_speed : Inport
  Vehicle_speed_target : Inport  Port=2
  Distance_m : Inport  Port=3
  dT : Inport  Port=4
  Detect Change1 : simulink/Logic and Bit Operations/Detect Change  vinit=0  InputProcessing=Inherited  OutDataTypeStr=boolean
      settings: AttributesFormatString=IC: %<vinit>
  Determine_slew_time_values : Subsystem
  Logical Operator : EmE_MBD_Blockset/Logic and Bit Operations/Logical Operator  Operator=OR  Inputs=1
      settings: SourceProductName=PACCAR EmE MBD Blockset
  Mux : Mux  Inputs=2
  Slew_init_reset : EmE_MBD_Blockset/Math Operators/Slew_init_reset
      settings: SourceProductName=PACCAR EmE MBD Blockset
  Vehicle_speed_profile_linear : Outport  OutputWhenDisabled=reset
  wires:
  dT/1 -> Slew_init_reset/6, Determine_slew_time_values/5(dT)
  Slew_init_reset/1 -> Vehicle_speed_profile_linear/1  "Vehicle_speed_profile_linear"
  Detect Change1/1 -> Logical Operator/1
  Mux/1 -> Detect Change1/1
  Logical Operator/1 -> Determine_slew_time_values/1(F_Reset), Slew_init_reset/1
  Vehicle_speed_target/1 -> Determine_slew_time_values/3(Vehicle_speed_target), Slew_init_reset/3, Mux/2
  Distance_m/1 -> Determine_slew_time_values/4(Distance_m), Mux/1
  Vehicle_speed/1 -> Determine_slew_time_values/2(Vehicle_speed), Slew_init_reset/2
  Determine_slew_time_values/1(Inc) -> Slew_init_reset/4
  Determine_slew_time_values/2(Dec) -> Slew_init_reset/5

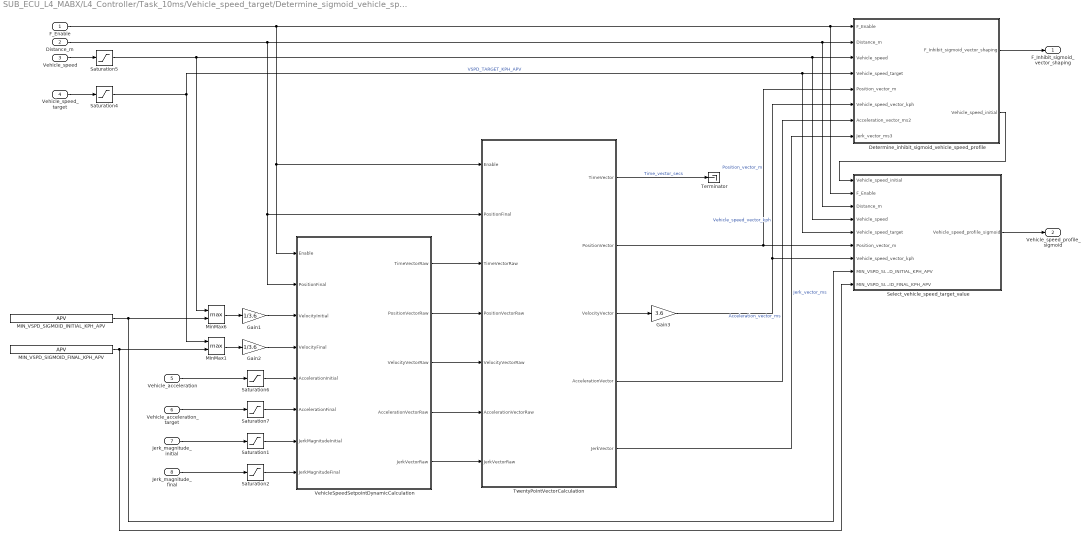
== system SUB_ECU_L4_MABX/L4_Controller/Task_10ms/Vehicle_speed_target/Determine_sigmoid_vehicle_speed_profile ==
  F_Enable : Inport
  Distance_m : Inport  Port=2
  Vehicle_speed : Inport  Port=3
  Vehicle_speed_target : Inport  Port=4
  Vehicle_acceleration : Inport  Port=5
  Vehicle_acceleration_target : Inport  Port=6
  Jerk_magnitude_initial : Inport  Port=7
  Jerk_magnitude_final : Inport  Port=8
  Determine_inhibit_sigmoid_vehicle_speed_profile : Subsystem
  Gain1 : Gain  Gain=1/3.6
  Gain2 : Gain  Gain=1/3.6
  Gain3 : Gain  Gain=3.6
  MIN_VSPD_SIGMOID_FINAL_KPH_APV : EmE_MBD_Blockset/Sources/APV  conval=0
      settings: SourceProductName=PACCAR EmE MBD Blockset
  MIN_VSPD_SIGMOID_INITIAL_KPH_APV : EmE_MBD_Blockset/Sources/APV  conval=5
      settings: SourceProductName=PACCAR EmE MBD Blockset
  MinMax1 : MinMax  Function=max  Inputs=2  InputSameDT=on
  MinMax6 : MinMax  Function=max  Inputs=2  InputSameDT=on
  Saturation1 : Saturate  UpperLimit=10  LowerLimit=0.001
      settings: AttributesFormatString=|
      | Min: %<LowerLimit>
      | Max: %<UpperLimit>
  Saturation2 : Saturate  UpperLimit=10  LowerLimit=0.001
      settings: AttributesFormatString=|
      | Min: %<LowerLimit>
      | Max: %<UpperLimit>
  Saturation4 : Saturate  UpperLimit=255  LowerLimit=0
      settings: AttributesFormatString=|
      | Min: %<LowerLimit>
      | Max: %<UpperLimit>
  Saturation5 : Saturate  UpperLimit=255  LowerLimit=0
      settings: AttributesFormatString=|
      | Min: %<LowerLimit>
      | Max: %<UpperLimit>
  Saturation6 : Saturate  UpperLimit=15.562  LowerLimit=-15.562
      settings: AttributesFormatString=|
      | Min: %<LowerLimit>
      | Max: %<UpperLimit>
  Saturation7 : Saturate  UpperLimit=15.562  LowerLimit=-15.562
      settings: AttributesFormatString=|
      | Min: %<LowerLimit>
      | Max: %<UpperLimit>
  Select_vehicle_speed_target_value : Subsystem
  Terminator : Terminator
  TwentyPointVectorCalculation : Stateflow chart  TreatAsAtomicUnit=on
  VehicleSpeedSetpointDynamicCalculation : Stateflow chart  TreatAsAtomicUnit=on
  F_Inhibit_sigmoid_vector_shaping : Outport  LibraryBlock=EmE_MBD_Blockset/Sinks/Out  OutputWhenDisabled=reset
  Vehicle_speed_profile_sigmoid : Outport  Port=2
  wires:
  Saturation2/1 -> VehicleSpeedSetpointDynamicCalculation/8(JerkMagnitudeFinal)
  Saturation1/1 -> VehicleSpeedSetpointDynamicCalculation/7(JerkMagnitudeInitial)
  Saturation7/1 -> VehicleSpeedSetpointDynamicCalculation/6(AccelerationFinal)
  Saturation6/1 -> VehicleSpeedSetpointDynamicCalculation/5(AccelerationInitial)
  Vehicle_speed_target/1 -> Saturation4/1
  Saturation5/1 -> Determine_inhibit_sigmoid_vehicle_speed_profile/3(Vehicle_speed), Select_vehicle_speed_target_value/4(Vehicle_speed), MinMax6/1
  Saturation4/1 -> Determine_inhibit_sigmoid_vehicle_speed_profile/4(Vehicle_speed_target), Select_vehicle_speed_target_value/5(Vehicle_speed_target), MinMax1/1  "VSPD_TARGET_KPH_APV"
  Determine_inhibit_sigmoid_vehicle_speed_profile/2(Vehicle_speed_initial) -> Select_vehicle_speed_target_value/1(Vehicle_speed_initial)
  MinMax6/1 -> Gain1/1
  MinMax1/1 -> Gain2/1
  MIN_VSPD_SIGMOID_FINAL_KPH_APV/1 -> Select_vehicle_speed_target_value/9(MIN_VSPD_SIGMOID_FINAL_KPH_APV), MinMax1/2
  MIN_VSPD_SIGMOID_INITIAL_KPH_APV/1 -> Select_vehicle_speed_target_value/8(MIN_VSPD_SIGMOID_INITIAL_KPH_APV), MinMax6/2
  Jerk_magnitude_final/1 -> Saturation2/1
  Jerk_magnitude_initial/1 -> Saturation1/1
  VehicleSpeedSetpointDynamicCalculation/3(VelocityVectorRaw) -> TwentyPointVectorCalculation/5(VelocityVectorRaw)
  TwentyPointVectorCalculation/2(PositionVector) -> Select_vehicle_speed_target_value/6(Position_vector_m), Determine_inhibit_sigmoid_vehicle_speed_profile/5(Position_vector_m)  "Position_vector_m"
  VehicleSpeedSetpointDynamicCalculation/1(TimeVectorRaw) -> TwentyPointVectorCalculation/3(TimeVectorRaw)
  TwentyPointVectorCalculation/5(JerkVector) -> Determine_inhibit_sigmoid_vehicle_speed_profile/8(Jerk_vector_ms3)  "Jerk_vector_ms"
  VehicleSpeedSetpointDynamicCalculation/2(PositionVectorRaw) -> TwentyPointVectorCalculation/4(PositionVectorRaw)
  TwentyPointVectorCalculation/4(AccelerationVector) -> Determine_inhibit_sigmoid_vehicle_speed_profile/7(Acceleration_vector_ms2)  "Acceleration_vector_ms"
  VehicleSpeedSetpointDynamicCalculation/4(AccelerationVectorRaw) -> TwentyPointVectorCalculation/6(AccelerationVectorRaw)
  TwentyPointVectorCalculation/3(VelocityVector) -> Gain3/1
  TwentyPointVectorCalculation/1(TimeVector) -> Terminator/1  "Time_vector_secs"
  VehicleSpeedSetpointDynamicCalculation/5(JerkVectorRaw) -> TwentyPointVectorCalculation/7(JerkVectorRaw)
  Select_vehicle_speed_target_value/1(Vehicle_speed_profile_sigmoid) -> Vehicle_speed_profile_sigmoid/1
  Vehicle_speed/1 -> Saturation5/1
  Determine_inhibit_sigmoid_vehicle_speed_profile/1(F_Inhibit_sigmoid_vector_shaping) -> F_Inhibit_sigmoid_vector_shaping/1
  Vehicle_acceleration_target/1 -> Saturation7/1
  Gain3/1 -> Select_vehicle_speed_target_value/7(Vehicle_speed_vector_kph), Determine_inhibit_sigmoid_vehicle_speed_profile/6(Vehicle_speed_vector_kph)  "Vehicle_speed_vector_kph"
  Vehicle_acceleration/1 -> Saturation6/1
  Gain1/1 -> VehicleSpeedSetpointDynamicCalculation/3(VelocityInitial)
  Gain2/1 -> VehicleSpeedSetpointDynamicCalculation/4(VelocityFinal)
  Distance_m/1 -> Determine_inhibit_sigmoid_vehicle_speed_profile/2(Distance_m), Select_vehicle_speed_target_value/3(Distance_m), TwentyPointVectorCalculation/2(PositionFinal), VehicleSpeedSetpointDynamicCalculation/2(PositionFinal)
  F_Enable/1 -> Determine_inhibit_sigmoid_vehicle_speed_profile/1(F_Enable), Select_vehicle_speed_target_value/2(F_Enable), TwentyPointVectorCalculation/1(Enable), VehicleSpeedSetpointDynamicCalculation/1(Enable)

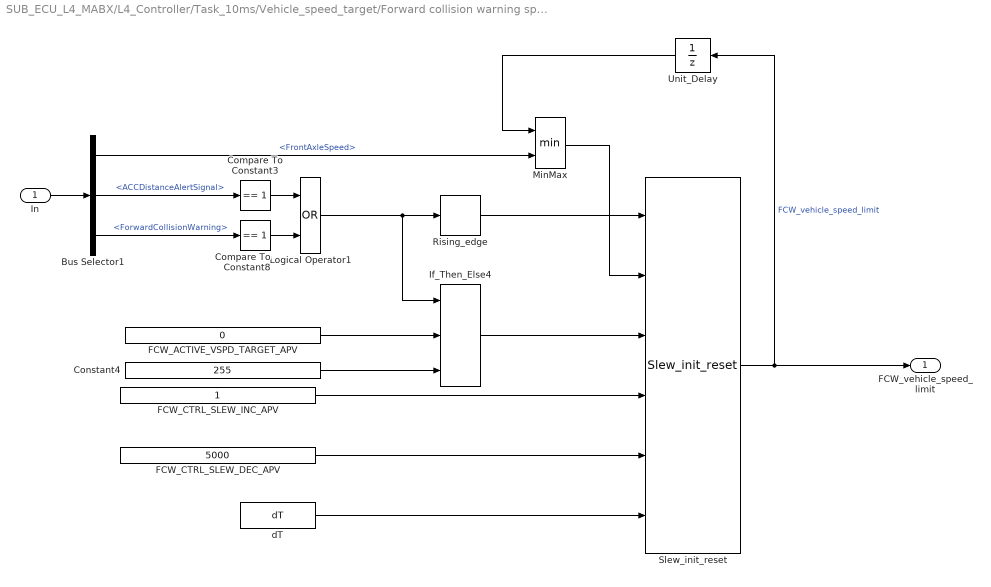
== system SUB_ECU_L4_MABX/L4_Controller/Task_10ms/Vehicle_speed_target/Forward collision warning speed limit ==
  In : Inport
  Bus Selector1 : BusSelector  OutputSignals=CAN.EBC2_0B.FrontAxleSpeed,CAN.ACC1_2A.ACCDistanceAlertSignal,CAN.ACC1_2A.ForwardCollisionWarning
  Compare To Constant3 : simulink/Logic and Bit Operations/Compare To Constant  relop===  const=1  OutDataTypeStr=boolean
  Compare To Constant8 : simulink/Logic and Bit Operations/Compare To Constant  relop===  const=1  OutDataTypeStr=boolean
  Constant4 : Constant  Value=255
  FCW_ACTIVE_VSPD_TARGET_APV : Constant  Value=0
  FCW_CTRL_SLEW_DEC_APV : Constant  Value=5000
  FCW_CTRL_SLEW_INC_APV : Constant
  If_Then_Else4 : EmE_MBD_Blockset/Signal Routing/If_Then_Else
      settings: SourceProductName=PACCAR EmE MBD Blockset
  Logical Operator1 : Logic  Operator=OR  OutDataTypeStr=boolean
  MinMax : MinMax  Inputs=2  InputSameDT=on
  Rising_edge : EmE_MBD_Blockset/Discontinuities/Rising_edge  initact=off
      settings: AttributesFormatString=Action on IC: %<initact>  SourceProductName=PACCAR EmE MBD Blockset
  Slew_init_reset : EmE_MBD_Blockset/Math Operators/Slew_init_reset
      settings: SourceProductName=PACCAR EmE MBD Blockset
  Unit_Delay : UnitDelay  SampleTime=-1
      settings: AttributesFormatString=IC: %<vinit>
  dT : EmE_MBD_Blockset/Sources/dT
      settings: SourceProductName=PACCAR EmE MBD Blockset
  FCW_vehicle_speed_limit : Outport
  wires:
  In/1 -> Bus Selector1/1
  Compare To Constant3/1 -> Logical Operator1/1
  Bus Selector1/2 -> Compare To Constant3/1  "<ACCDistanceAlertSignal>"
  Compare To Constant8/1 -> Logical Operator1/2
  Bus Selector1/3 -> Compare To Constant8/1  "<ForwardCollisionWarning>"
  Rising_edge/1 -> Slew_init_reset/1
  Unit_Delay/1 -> MinMax/1
  If_Then_Else4/1 -> Slew_init_reset/3
  Logical Operator1/1 -> If_Then_Else4/1, Rising_edge/1
  dT/1 -> Slew_init_reset/6
  Constant4/1 -> If_Then_Else4/3
  Bus Selector1/1 -> MinMax/2  "<FrontAxleSpeed>"
  Slew_init_reset/1 -> FCW_vehicle_speed_limit/1, Unit_Delay/1  "FCW_vehicle_speed_limit"
  FCW_CTRL_SLEW_DEC_APV/1 -> Slew_init_reset/5
  FCW_ACTIVE_VSPD_TARGET_APV/1 -> If_Then_Else4/2
  FCW_CTRL_SLEW_INC_APV/1 -> Slew_init_reset/4
  MinMax/1 -> Slew_init_reset/2

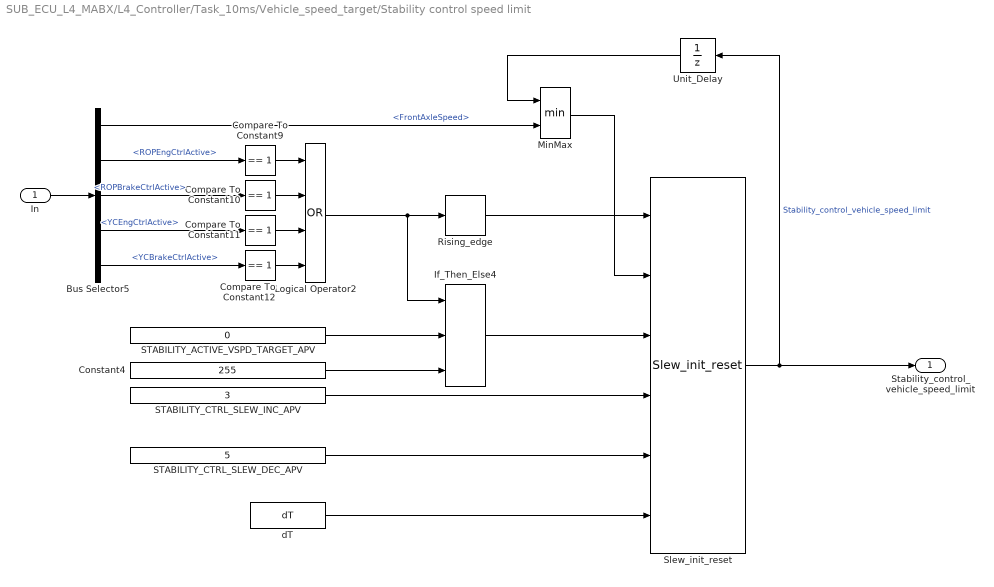
== system SUB_ECU_L4_MABX/L4_Controller/Task_10ms/Vehicle_speed_target/Stability control speed limit ==
  In : Inport
  Bus Selector5 : BusSelector  OutputSignals=CAN.EBC2_0B.FrontAxleSpeed,CAN.VDC1_0B.ROPEngCtrlActive,CAN.VDC1_0B.ROPBrakeCtrlActive,CAN.VDC1_0B.YCEngCtrlActive,CAN.VDC1_0B.YCBrakeCtrlActive
  Compare To Constant{9..12} (4 alike) : simulink/Logic and Bit Operations/Compare To Constant  relop===  const=1  OutDataTypeStr=boolean
  Constant4 : Constant  Value=255
  If_Then_Else4 : EmE_MBD_Blockset/Signal Routing/If_Then_Else
      settings: SourceProductName=PACCAR EmE MBD Blockset
  Logical Operator2 : Logic  Operator=OR  Inputs=4  OutDataTypeStr=boolean
  MinMax : MinMax  Inputs=2  InputSameDT=on
  Rising_edge : EmE_MBD_Blockset/Discontinuities/Rising_edge  initact=off
      settings: AttributesFormatString=Action on IC: %<initact>  SourceProductName=PACCAR EmE MBD Blockset
  STABILITY_ACTIVE_VSPD_TARGET_APV : Constant  Value=0
  STABILITY_CTRL_SLEW_DEC_APV : Constant  Value=5
  STABILITY_CTRL_SLEW_INC_APV : Constant  Value=3
  Slew_init_reset : EmE_MBD_Blockset/Math Operators/Slew_init_reset
      settings: SourceProductName=PACCAR EmE MBD Blockset
  Unit_Delay : UnitDelay  SampleTime=-1
      settings: AttributesFormatString=IC: %<vinit>
  dT : EmE_MBD_Blockset/Sources/dT
      settings: SourceProductName=PACCAR EmE MBD Blockset
  Stability_control_vehicle_speed_limit : Outport
  wires:
  Bus Selector5/4 -> Compare To Constant11/1  "<YCEngCtrlActive>"
  Bus Selector5/2 -> Compare To Constant9/1  "<ROPEngCtrlActive>"
  Bus Selector5/5 -> Compare To Constant12/1  "<YCBrakeCtrlActive>"
  Compare To Constant10/1 -> Logical Operator2/2
  Compare To Constant12/1 -> Logical Operator2/4
  Compare To Constant9/1 -> Logical Operator2/1
  Compare To Constant11/1 -> Logical Operator2/3
  dT/1 -> Slew_init_reset/6
  Constant4/1 -> If_Then_Else4/3
  STABILITY_CTRL_SLEW_INC_APV/1 -> Slew_init_reset/4
  STABILITY_CTRL_SLEW_DEC_APV/1 -> Slew_init_reset/5
  STABILITY_ACTIVE_VSPD_TARGET_APV/1 -> If_Then_Else4/2
  If_Then_Else4/1 -> Slew_init_reset/3
  In/1 -> Bus Selector5/1
  Bus Selector5/3 -> Compare To Constant10/1  "<ROPBrakeCtrlActive>"
  Logical Operator2/1 -> If_Then_Else4/1, Rising_edge/1
  Slew_init_reset/1 -> Stability_control_vehicle_speed_limit/1, Unit_Delay/1  "Stability_control_vehicle_speed_limit"
  Rising_edge/1 -> Slew_init_reset/1
  MinMax/1 -> Slew_init_reset/2
  Bus Selector5/1 -> MinMax/2  "<FrontAxleSpeed>"
  Unit_Delay/1 -> MinMax/1

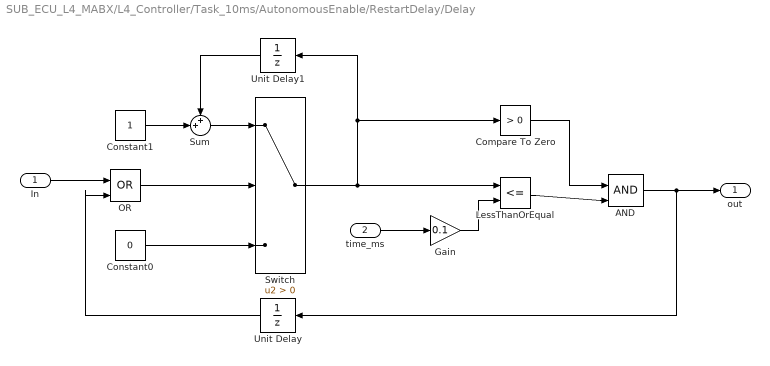
== system SUB_ECU_L4_MABX/L4_Controller/Task_10ms/AutonomousEnable/RestartDelay/Delay ==
  In : Inport
  time_ms : Inport  Port=2
  AND : Logic  IconShape=distinctive  AllPortsSameDT=off  OutDataTypeStr=boolean
  Compare To Zero : simulink/Logic and Bit Operations/Compare To Zero  relop=>  OutDataTypeStr=boolean
  Constant0 : Constant  Value=0
  Constant1 : Constant
  Gain : Gain  Gain=0.1
  LessThanOrEqual : RelationalOperator  Operator=<=  OutDataTypeStr=boolean  RndMeth=Simplest
  OR : Logic  Operator=OR  IconShape=distinctive  AllPortsSameDT=off  OutDataTypeStr=boolean
  Sum : Sum  Inputs=++|
  Switch : Switch  Criteria=u2 > Threshold
  Unit Delay : UnitDelay  SampleTime=-1
  Unit Delay1 : UnitDelay  SampleTime=-1
  out : Outport
  wires:
  time_ms/1 -> Gain/1
  Gain/1 -> LessThanOrEqual/2
  Constant1/1 -> Sum/2
  Unit Delay1/1 -> Sum/1
  OR/1 -> Switch/2
  Constant0/1 -> Switch/3
  In/1 -> OR/1
  Unit Delay/1 -> OR/2
  Sum/1 -> Switch/1
  LessThanOrEqual/1 -> AND/2
  Compare To Zero/1 -> AND/1
  AND/1 -> out/1, Unit Delay/1
  Switch/1 -> Unit Delay1/1, Compare To Zero/1, LessThanOrEqual/1

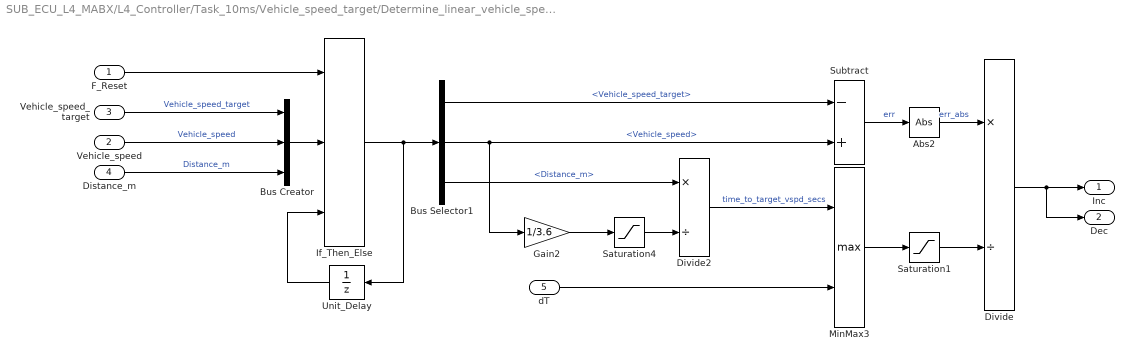
== system SUB_ECU_L4_MABX/L4_Controller/Task_10ms/Vehicle_speed_target/Determine_linear_vehicle_speed_profile/Determine_slew_time_values ==
  F_Reset : Inport
  Vehicle_speed : Inport  Port=2
  Vehicle_speed_target : Inport  Port=3
  Distance_m : Inport  Port=4
  dT : Inport  Port=5
  Abs2 : EmE_MBD_Blockset/Math Operators/Abs
      settings: SourceProductName=PACCAR EmE MBD Blockset
  Bus Creator : BusCreator  Inputs=3
  Bus Selector1 : BusSelector  OutputSignals=Vehicle_speed_target,Vehicle_speed,Distance_m
  Divide : Product  Inputs=*/  InputSameDT=on
  Divide2 : Product  Inputs=*/  InputSameDT=on
  Gain2 : Gain  Gain=1/3.6
  If_Then_Else : EmE_MBD_Blockset/Signal Routing/If_Then_Else
      settings: SourceProductName=PACCAR EmE MBD Blockset
  MinMax3 : MinMax  Function=max  Inputs=2  InputSameDT=on
  Saturation1 : Saturate  UpperLimit=Inf  LowerLimit=0.001
      settings: AttributesFormatString=|
      | Min: %<LowerLimit>
      | Max: %<UpperLimit>
  Saturation4 : Saturate  UpperLimit=255  LowerLimit=0.001
      settings: AttributesFormatString=|
      | Min: %<LowerLimit>
      | Max: %<UpperLimit>
  Subtract : Sum  Inputs=-+  InputSameDT=on
  Unit_Delay : UnitDelay  SampleTime=-1
      settings: AttributesFormatString=IC: %<vinit>
  Inc : Outport
  Dec : Outport  Port=2
  wires:
  Bus Selector1/2 -> Gain2/1, Subtract/2  "<Vehicle_speed>"
  Bus Selector1/3 -> Divide2/1  "<Distance_m>"
  Subtract/1 -> Abs2/1  "err"
  Gain2/1 -> Saturation4/1
  Divide2/1 -> MinMax3/1  "time_to_target_vspd_secs"
  Bus Selector1/1 -> Subtract/1  "<Vehicle_speed_target>"
  dT/1 -> MinMax3/2
  Saturation4/1 -> Divide2/2
  MinMax3/1 -> Saturation1/1
  Abs2/1 -> Divide/1  "err_abs"
  Divide/1 -> Dec/1, Inc/1
  Saturation1/1 -> Divide/2
  Bus Creator/1 -> If_Then_Else/2
  If_Then_Else/1 -> Unit_Delay/1, Bus Selector1/1
  Unit_Delay/1 -> If_Then_Else/3
  Distance_m/1 -> Bus Creator/3  "Distance_m"
  Vehicle_speed_target/1 -> Bus Creator/1  "Vehicle_speed_target"
  Vehicle_speed/1 -> Bus Creator/2  "Vehicle_speed"
  F_Reset/1 -> If_Then_Else/1
